simulink model "gm_sampleModel1495_sub"  (R2023a)
settings: Solver=VariableStepAuto  StartTime=0.0  StopTime=10.0  RelTol=1e-3
libraries: hdlsllib x3
settings Model: Creator=user1  LastModifiedBy=user1
settings OptimizationCC: BlockReduction=off  ConditionallyExecuteInputs=off
settings DebuggingCC: InheritedTsInSrcMsg=none

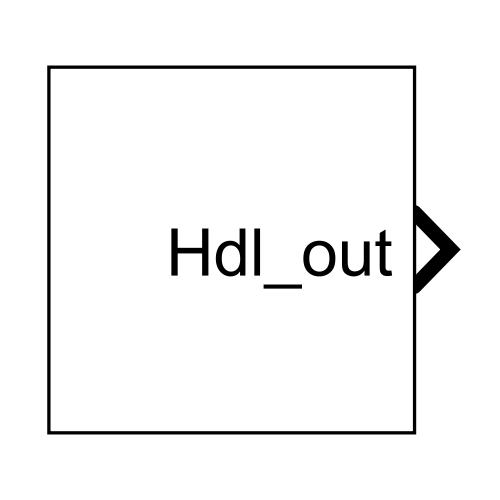
[thumbnail: Simulink's stored preview of the top-level diagram]
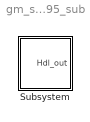
== system gm_sampleModel1495_sub ==
  Subsystem : Subsystem

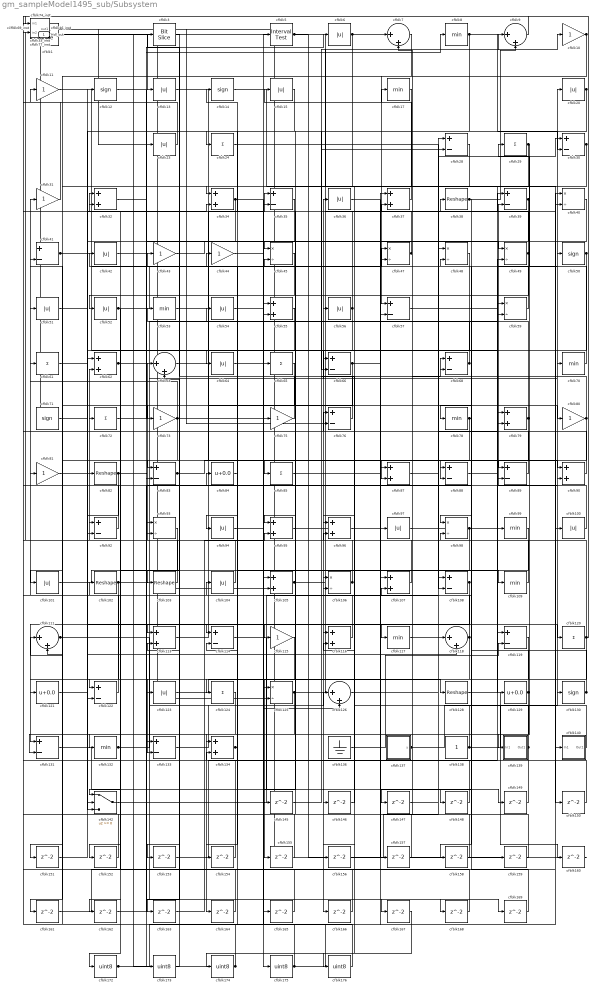
== system gm_sampleModel1495_sub/Subsystem ==
  cfblk1 : hdlsllib/Logic and Bit Operations/Bit Slice  lidx=7  ridx=0
  cfblk{10..11,31,43..44,73,75,80..81,115} (10 alike) : Gain  OutDataTypeStr=uint8
  cfblk{6,13,15,20,23,36,42,51..52,54,56,64,94,97,100..101,104,123} (18 alike) : Abs  OutDataTypeStr=uint8  SaturateOnIntegerOverflow=off
  cfblk{38,82,102..103,128} (5 alike) : Reshape
  cfblk{32,34,37,55,62,79,87,90,95..96,105,107,113,116,134} (15 alike) : Sum  OutDataTypeStr=uint8
  cfblk{40,45,47..49,59,93,98,106,125} (10 alike) : Product  Inputs=*/  OutDataTypeStr=uint8  RndMeth=Zero  SaturateOnIntegerOverflow=on
  cfblk{28,30,35,39,41,57,66,68,76,83,88..89,92,108,114,119,122,131,133} (19 alike) : Sum  Inputs=+-  OutDataTypeStr=uint8
  cfblk{8,17,53,70,78,99,109,117,132} (9 alike) : MinMax  OutDataTypeStr=uint8
  cfblk110_inst : Subsystem
  cfblk{7,9,63,111,118,126} (6 alike) : Sum  Inputs=|++  OutDataTypeStr=uint8
  cfblk{12,14,50,71,130} (5 alike) : Signum
  cfblk{24,29,61,65,72,85,120,124} (8 alike) : Sum  Inputs=+  OutDataTypeStr=uint8
  cfblk121 : Bias  Bias=0.0  SaturateOnIntegerOverflow=off
  cfblk129 : Bias  Bias=0.0  SaturateOnIntegerOverflow=off
  cfblk136 : Ground
  cfblk137 : Subsystem  mask(Counter Free-Running){NumBits=double(16), tsamp=double(-1)}
      mask prompts: NumBits "Simulink:masks:NumberOfBits_MP"; tsamp "Simulink:masks:SampleTime_MP"
      mask help: Simulink:masks:CounterFreeRunning_MD
  cfblk138 : Constant  OutDataTypeStr=uint8  SampleTime=-1
  cfblk139 : Subsystem
  cfblk140 : Subsystem
  cfblk142 : Switch  OutDataTypeStr=uint8  SaturateOnIntegerOverflow=off  InputSameDT=off
  cfblk{145..169} (25 alike) : Delay  SampleTime=1
  cfblk16_inst : Subsystem
  cfblk{172..176} (5 alike) : DataTypeConversion  OutDataTypeStr=uint8  SaturateOnIntegerOverflow=off  RndMeth=Floor
  cfblk21_inst : Subsystem
  cfblk3 : hdlsllib/Logic and Bit Operations/Bit Slice  lidx=7  ridx=0
  cfblk33_inst : Subsystem
  cfblk46_inst : Subsystem
  cfblk5 : hdlsllib/Logic and Bit Operations/Interval Test  IntervalClosedRight=on  uplimit=0.5  IntervalClosedLeft=on  lowlimit=-0.5  OutDataTypeStr=uint8
  cfblk69_inst : Subsystem
  cfblk74_inst : Subsystem
  cfblk77_inst : Subsystem
  cfblk84 : Bias  Bias=0.0  SaturateOnIntegerOverflow=off
  Hdl_out : Outport  OutDataTypeStr=uint8  SampleTime=1
  wires:
  cfblk1/1 -> cfblk13/1
  cfblk10/1 -> cfblk57/1, cfblk111/2
  cfblk100/1 -> cfblk39/2
  cfblk101/1 -> cfblk109/1
  cfblk102/1 -> cfblk122/1, cfblk59/2, cfblk152/1
  cfblk103/1 -> cfblk63/1
  cfblk104/1 -> cfblk110_inst/2(in2)
  cfblk105/1 -> cfblk9/1, cfblk38/1
  cfblk106/1 -> cfblk16_inst/2(in2), cfblk31/1
  cfblk107/1 -> cfblk62/2
  cfblk108/1 -> cfblk131/1, cfblk117/1
  cfblk109/1 -> cfblk72/1
  cfblk11/1 -> cfblk166/1
  cfblk110_inst/1(out1) -> cfblk105/2
  cfblk111/1 -> cfblk20/1, cfblk167/1
  cfblk113/1 -> cfblk35/1
  cfblk114/1 -> cfblk146/1
  cfblk115/1 -> cfblk161/1
  cfblk116/1 -> cfblk102/1
  cfblk117/1 -> cfblk28/1
  cfblk118/1 -> cfblk51/1, cfblk133/2
  cfblk119/1 -> cfblk147/1
  cfblk12/1 -> cfblk168/1
  cfblk120/1 -> cfblk33_inst/1(in1), cfblk98/2, cfblk155/1
  cfblk121/1 -> cfblk118/2
  cfblk122/1 -> cfblk77_inst/1(in1)
  cfblk123/1 -> cfblk128/1
  cfblk124/1 -> cfblk164/1
  cfblk125/1 -> cfblk131/2, cfblk59/1
  cfblk126/1 -> cfblk79/2
  cfblk128/1 -> cfblk160/1
  cfblk129/1 -> cfblk43/1, cfblk163/1, cfblk124/1
  cfblk13/1 -> cfblk87/2
  cfblk130/1 -> cfblk105/1, cfblk81/1
  cfblk131/1 -> cfblk149/1
  cfblk132/1 -> cfblk36/1, cfblk126/1
  cfblk133/1 -> cfblk10/1
  cfblk134/1 -> cfblk84/1, cfblk114/2
  cfblk136/1 -> cfblk119/2
  cfblk137/1(y) -> cfblk79/1, cfblk70/1
  cfblk138/1 -> cfblk130/1, cfblk104/1
  cfblk139/1(Out1) -> cfblk134/2, cfblk116/2
  cfblk14/1 -> cfblk100/1
  cfblk140/1(Out1) -> cfblk66/1
  cfblk142/1 -> cfblk48/1
  cfblk145/1 -> cfblk28/2
  cfblk146/1 -> cfblk76/1
  cfblk147/1 -> cfblk108/1
  cfblk148/1 -> cfblk74_inst/2(in2)
  cfblk149/1 -> cfblk37/2
  cfblk15/1 -> cfblk24/1
  cfblk150/1 -> cfblk111/1
  cfblk151/1 -> cfblk34/2
  cfblk152/1 -> cfblk62/1
  cfblk153/1 -> cfblk49/2
  cfblk154/1 -> cfblk46_inst/1(in1)
  cfblk155/1 -> cfblk69_inst/1(in1)
  cfblk156/1 -> cfblk118/1
  cfblk157/1 -> cfblk35/2
  cfblk158/1 -> cfblk32/1
  cfblk159/1 -> cfblk107/2
  cfblk16_inst/1(out1) -> cfblk71/1, cfblk125/2
  cfblk160/1 -> cfblk1/1
  cfblk161/1 -> cfblk40/2
  cfblk162/1 -> cfblk90/2
  cfblk163/1 -> cfblk95/2
  cfblk164/1 -> cfblk63/2
  cfblk165/1 -> cfblk113/2
  cfblk166/1 -> cfblk92/1
  cfblk167/1 -> cfblk174/1
  cfblk168/1 -> cfblk21_inst/1(in1)
  cfblk169/1 -> cfblk68/1
  cfblk17/1 -> cfblk94/1
  cfblk172/1 -> cfblk140/1(In1), cfblk65/1
  cfblk173/1 -> cfblk93/1
  cfblk174/1 -> cfblk93/2, Hdl_out/1
  cfblk175/1 -> cfblk87/1, cfblk77_inst/2(in2), cfblk41/2
  cfblk176/1 -> cfblk44/1
  cfblk20/1 -> cfblk66/2, cfblk145/1
  cfblk21_inst/1(out1) -> cfblk76/2
  cfblk23/1 -> cfblk21_inst/2(in2)
  cfblk24/1 -> cfblk90/1
  cfblk28/1 -> cfblk113/1
  cfblk29/1 -> cfblk176/1, cfblk139/1(In1)
  cfblk3/1 -> cfblk153/1
  cfblk30/1 -> cfblk106/2, cfblk106/1
  cfblk31/1 -> cfblk11/1
  cfblk32/1 -> cfblk173/1
  cfblk33_inst/1(out1) -> cfblk75/1, cfblk99/1
  cfblk34/1 -> cfblk55/2, cfblk103/1
  cfblk35/1 -> cfblk92/2
  cfblk36/1 -> cfblk97/1
  cfblk37/1 -> cfblk15/1
  cfblk38/1 -> cfblk9/2, cfblk158/1
  cfblk39/1 -> cfblk88/2, cfblk114/1
  cfblk40/1 -> cfblk95/1
  cfblk41/1 -> cfblk129/1, cfblk45/2, cfblk165/1
  cfblk42/1 -> cfblk45/1
  cfblk43/1 -> cfblk49/1
  cfblk44/1 -> cfblk175/1
  cfblk45/1 -> cfblk83/1
  cfblk46_inst/1(out1) -> cfblk41/1
  cfblk47/1 -> cfblk33_inst/2(in2), cfblk17/1
  cfblk48/1 -> cfblk125/1
  cfblk49/1 -> cfblk7/2, cfblk57/2, cfblk52/1, cfblk48/2
  cfblk5/1 -> cfblk89/2, cfblk150/1
  cfblk50/1 -> cfblk96/1, cfblk78/1
  cfblk51/1 -> cfblk12/1
  cfblk52/1 -> cfblk142/1, cfblk5/1
  cfblk53/1 -> cfblk107/1
  cfblk54/1 -> cfblk148/1
  cfblk55/1 -> cfblk123/1
  cfblk56/1 -> cfblk142/2, cfblk14/1
  cfblk57/1 -> cfblk50/1
  cfblk59/1 -> cfblk42/1
  cfblk6/1 -> cfblk7/1, cfblk121/1
  cfblk61/1 -> cfblk115/1
  cfblk62/1 -> cfblk83/2, cfblk8/1
  cfblk63/1 -> cfblk80/1
  cfblk64/1 -> cfblk169/1
  cfblk65/1 -> cfblk101/1
  cfblk66/1 -> cfblk37/1, cfblk132/1
  cfblk68/1 -> cfblk64/1, cfblk53/1
  cfblk69_inst/1(out1) -> cfblk23/1
  cfblk7/1 -> cfblk73/1
  cfblk70/1 -> cfblk29/1
  cfblk71/1 -> cfblk120/1
  cfblk72/1 -> cfblk6/1
  cfblk73/1 -> cfblk47/1, cfblk151/1, cfblk61/1
  cfblk74_inst/1(out1) -> cfblk46_inst/2(in2)
  cfblk75/1 -> cfblk3/1
  cfblk76/1 -> cfblk32/2
  cfblk77_inst/1(out1) -> cfblk110_inst/1(in1), cfblk159/1
  cfblk78/1 -> cfblk98/1, cfblk162/1
  cfblk79/1 -> cfblk56/1, cfblk55/1, cfblk116/1
  cfblk8/1 -> cfblk34/1, cfblk30/2, cfblk142/3
  cfblk80/1 -> cfblk108/2, cfblk47/2
  cfblk81/1 -> cfblk82/1
  cfblk82/1 -> cfblk133/1, cfblk122/2
  cfblk83/1 -> cfblk89/1, cfblk88/1, cfblk85/1
  cfblk84/1 -> cfblk154/1
  cfblk85/1 -> cfblk39/1
  cfblk87/1 -> cfblk40/1
  cfblk88/1 -> cfblk119/1
  cfblk89/1 -> cfblk54/1
  cfblk9/1 -> cfblk16_inst/1(in1)
  cfblk90/1 -> cfblk74_inst/1(in1)
  cfblk92/1 -> cfblk69_inst/2(in2)
  cfblk93/1 -> cfblk172/1
  cfblk94/1 -> cfblk126/2
  cfblk95/1 -> cfblk68/2
  cfblk96/1 -> cfblk157/1
  cfblk97/1 -> cfblk30/1
  cfblk98/1 -> cfblk96/2, cfblk156/1
  cfblk99/1 -> cfblk134/1

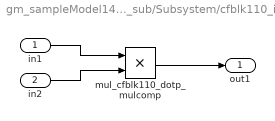
== system gm_sampleModel1495_sub/Subsystem/cfblk110_inst ==
  in1 : Inport  OutDataTypeStr=uint8  SampleTime=1
  in2 : Inport  Port=2  OutDataTypeStr=uint8  SampleTime=1
  mul_cfblk110_dotp_mulcomp : Product  Inputs=**  OutDataTypeStr=uint8  SampleTime=1
  out1 : Outport  OutDataTypeStr=uint8  SampleTime=1
  wires:
  in1/1 -> mul_cfblk110_dotp_mulcomp/1
  in2/1 -> mul_cfblk110_dotp_mulcomp/2
  mul_cfblk110_dotp_mulcomp/1 -> out1/1

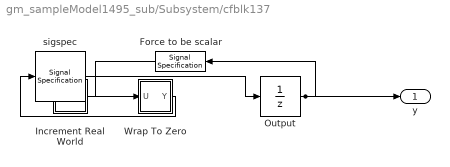
== system gm_sampleModel1495_sub/Subsystem/cfblk137 ==
  Force to be scalar : SignalSpecification  DisableCoverage=on  Dimensions=1
  Increment Real World : Subsystem  mask(Real World Value Increment){}
      mask help: Simulink:masks:RealWorldValueIncrement_MD
      mask Display: disp('V++')
  Output : UnitDelay  InitialCondition=0.0  SampleTime=tsamp  HasFrameUpgradeWarning=on
  Wrap To Zero : Subsystem  mask(Wrap To Zero){Threshold=double(65535)}
      mask prompts: Threshold "Simulink:masks:Threshold_MP"
      mask help: Simulink:masks:WrapToZero_MD
  sigspec : SignalSpecification  OutDataTypeStr=uint16  Dimensions=1
  y : Outport  SampleTime=1
  wires:
  Force to be scalar/1 -> Increment Real World/1(u)
  Increment Real World/1(y) -> Wrap To Zero/1(U)
  Output/1 -> Force to be scalar/1, y/1
  Wrap To Zero/1(Y) -> sigspec/1
  sigspec/1 -> Output/1

== system gm_sampleModel1495_sub/Subsystem/cfblk139 ==
  In1 : Inport  OutDataTypeStr=uint8  PortDimensions=1  SampleTime=1
  Out1 : Outport  SampleTime=1
  wires:
  In1/1 -> Out1/1

== system gm_sampleModel1495_sub/Subsystem/cfblk140 ==
  In1 : Inport  OutDataTypeStr=uint8  PortDimensions=1  SampleTime=1
  Out1 : Outport  SampleTime=1
  wires:
  In1/1 -> Out1/1

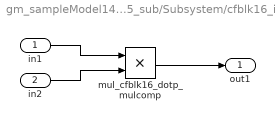
== system gm_sampleModel1495_sub/Subsystem/cfblk16_inst ==
  in1 : Inport  OutDataTypeStr=uint8  SampleTime=1
  in2 : Inport  Port=2  OutDataTypeStr=uint8  SampleTime=1
  mul_cfblk16_dotp_mulcomp : Product  Inputs=**  OutDataTypeStr=uint8  SampleTime=1
  out1 : Outport  OutDataTypeStr=uint8  SampleTime=1
  wires:
  in1/1 -> mul_cfblk16_dotp_mulcomp/1
  in2/1 -> mul_cfblk16_dotp_mulcomp/2
  mul_cfblk16_dotp_mulcomp/1 -> out1/1

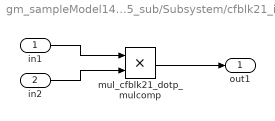
== system gm_sampleModel1495_sub/Subsystem/cfblk21_inst ==
  in1 : Inport  OutDataTypeStr=uint8  SampleTime=1
  in2 : Inport  Port=2  OutDataTypeStr=uint8  SampleTime=1
  mul_cfblk21_dotp_mulcomp : Product  Inputs=**  OutDataTypeStr=uint8  SampleTime=1
  out1 : Outport  OutDataTypeStr=uint8  SampleTime=1
  wires:
  in1/1 -> mul_cfblk21_dotp_mulcomp/1
  in2/1 -> mul_cfblk21_dotp_mulcomp/2
  mul_cfblk21_dotp_mulcomp/1 -> out1/1

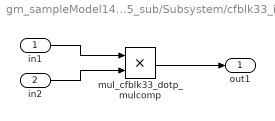
== system gm_sampleModel1495_sub/Subsystem/cfblk33_inst ==
  in1 : Inport  OutDataTypeStr=uint8  SampleTime=1
  in2 : Inport  Port=2  OutDataTypeStr=uint8  SampleTime=1
  mul_cfblk33_dotp_mulcomp : Product  Inputs=**  OutDataTypeStr=uint8  SampleTime=1
  out1 : Outport  OutDataTypeStr=uint8  SampleTime=1
  wires:
  in1/1 -> mul_cfblk33_dotp_mulcomp/1
  in2/1 -> mul_cfblk33_dotp_mulcomp/2
  mul_cfblk33_dotp_mulcomp/1 -> out1/1

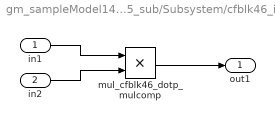
== system gm_sampleModel1495_sub/Subsystem/cfblk46_inst ==
  in1 : Inport  OutDataTypeStr=uint8  SampleTime=1
  in2 : Inport  Port=2  OutDataTypeStr=uint8  SampleTime=1
  mul_cfblk46_dotp_mulcomp : Product  Inputs=**  OutDataTypeStr=uint8  SampleTime=1
  out1 : Outport  OutDataTypeStr=uint8  SampleTime=1
  wires:
  in1/1 -> mul_cfblk46_dotp_mulcomp/1
  in2/1 -> mul_cfblk46_dotp_mulcomp/2
  mul_cfblk46_dotp_mulcomp/1 -> out1/1

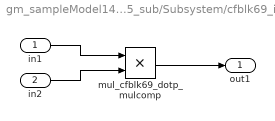
== system gm_sampleModel1495_sub/Subsystem/cfblk69_inst ==
  in1 : Inport  OutDataTypeStr=uint8  SampleTime=1
  in2 : Inport  Port=2  OutDataTypeStr=uint8  SampleTime=1
  mul_cfblk69_dotp_mulcomp : Product  Inputs=**  OutDataTypeStr=uint8  SampleTime=1
  out1 : Outport  OutDataTypeStr=uint8  SampleTime=1
  wires:
  in1/1 -> mul_cfblk69_dotp_mulcomp/1
  in2/1 -> mul_cfblk69_dotp_mulcomp/2
  mul_cfblk69_dotp_mulcomp/1 -> out1/1

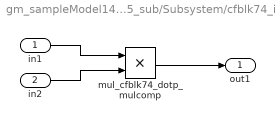
== system gm_sampleModel1495_sub/Subsystem/cfblk74_inst ==
  in1 : Inport  OutDataTypeStr=uint8  SampleTime=1
  in2 : Inport  Port=2  OutDataTypeStr=uint8  SampleTime=1
  mul_cfblk74_dotp_mulcomp : Product  Inputs=**  OutDataTypeStr=uint8  SampleTime=1
  out1 : Outport  OutDataTypeStr=uint8  SampleTime=1
  wires:
  in1/1 -> mul_cfblk74_dotp_mulcomp/1
  in2/1 -> mul_cfblk74_dotp_mulcomp/2
  mul_cfblk74_dotp_mulcomp/1 -> out1/1

== system gm_sampleModel1495_sub/Subsystem/cfblk77_inst ==
  in1 : Inport  OutDataTypeStr=uint8  SampleTime=1
  in2 : Inport  Port=2  OutDataTypeStr=uint8  SampleTime=1
  mul_cfblk77_dotp_mulcomp : Product  Inputs=**  OutDataTypeStr=uint8  SampleTime=1
  out1 : Outport  OutDataTypeStr=uint8  SampleTime=1
  wires:
  in1/1 -> mul_cfblk77_dotp_mulcomp/1
  in2/1 -> mul_cfblk77_dotp_mulcomp/2
  mul_cfblk77_dotp_mulcomp/1 -> out1/1

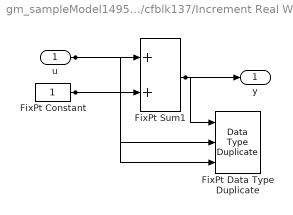
== system gm_sampleModel1495_sub/Subsystem/cfblk137/Increment Real World ==
  u : Inport  OutDataTypeStr=uint16  SampleTime=1
  FixPt Constant : Constant  DisableCoverage=on  OutDataTypeStr=Inherit: Inherit via back propagation  SampleTime=-1
  FixPt Data Type Duplicate : DataTypeDuplicate  DisableCoverage=on  NumInputPorts=3
  FixPt Sum1 : Sum  InputSameDT=on  OutDataTypeStr=Inherit: Inherit via back propagation  LockScale=on
  y : Outport  SampleTime=1
  wires:
  u/1 -> FixPt Sum1/1, FixPt Data Type Duplicate/2
  FixPt Constant/1 -> FixPt Sum1/2, FixPt Data Type Duplicate/3
  FixPt Sum1/1 -> FixPt Data Type Duplicate/1, y/1

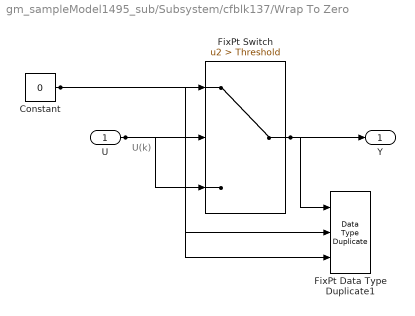
== system gm_sampleModel1495_sub/Subsystem/cfblk137/Wrap To Zero ==
  note: U(k)
  U : Inport  OutDataTypeStr=uint16  SampleTime=1
  Constant : Constant  DisableCoverage=on  Value=0  OutDataTypeStr=Inherit: Inherit via back propagation  SampleTime=-1
  FixPt Data Type Duplicate1 : DataTypeDuplicate  DisableCoverage=on  NumInputPorts=3
  FixPt Switch : Switch  Criteria=u2 > Threshold  Threshold=Threshold  OutDataTypeStr=Inherit: Inherit via back propagation  ZeroCross=off  SaturateOnIntegerOverflow=off  InputSameDT=off
  Y : Outport  SampleTime=1
  wires:
  U/1 -> FixPt Switch/3, FixPt Switch/2, FixPt Data Type Duplicate1/2
  Constant/1 -> FixPt Switch/1, FixPt Data Type Duplicate1/3
  FixPt Switch/1 -> FixPt Data Type Duplicate1/1, Y/1
